simulink model "lookuptable1D"  (Simulink 7.9)
settings: Solver=FixedStepDiscrete  StartTime=0.0  StopTime=10.0  FixedStep=1  RelTol=1e-3
settings Model: Creator=hnine  LastModifiedBy=hnine

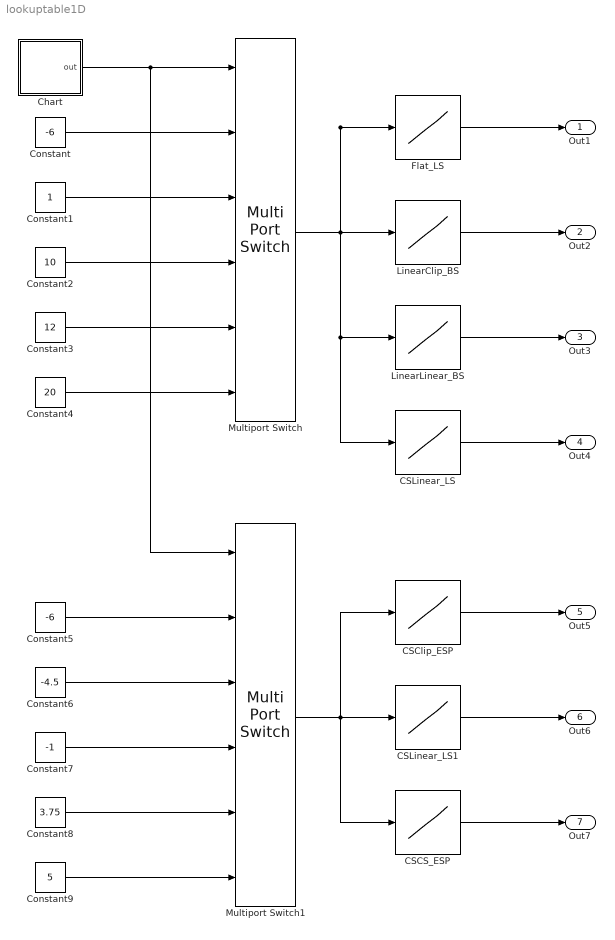
== system lookuptable1D ==
  CSCS_ESP : Lookup_n-D  NumberOfTableDimensions=1  BreakpointsForDimension1=[ -5 -4 -3 -2 -1 0 1 2 3 4 ]  IndexSearchMethod=Evenly spaced points  Table=[ 10 1 9 2 8 3 7 4 6 5 ]  InterpMethod=Cubic spline  ExtrapMethod=Cubic spline  RndMeth=Simplest  InputSameDT=on
  CSClip_ESP : Lookup_n-D  NumberOfTableDimensions=1  BreakpointsForDimension1=[ -5 -4 -3 -2 -1 0 1 2 3 4 ]  IndexSearchMethod=Evenly spaced points  Table=[ 10 1 9 2 8 3 7 4 6 5 ]  InterpMethod=Cubic spline  ExtrapMethod=Clip  RndMeth=Simplest  InputSameDT=on
  CSLinear_LS : Lookup_n-D  NumberOfTableDimensions=1  BreakpointsForDimension1=[ -4 -2 -0.5 .75 3 8 10 11 11.5 15 ]  IndexSearchMethod=Linear search  Table=[ 10 1 9 2 8 3 7 4 6 5 ]  InterpMethod=Cubic spline  RndMeth=Simplest  InputSameDT=on
  CSLinear_LS1 : Lookup_n-D  NumberOfTableDimensions=1  BreakpointsForDimension1=[ -5 -4 -3 -2 -1 0 1 2 3 4 ]  IndexSearchMethod=Linear search  Table=[ 10 1 9 2 8 3 7 4 6 5 ]  InterpMethod=Cubic spline  RndMeth=Simplest  InputSameDT=on
  Chart : Stateflow chart  TreatAsAtomicUnit=on
  Constant : Constant  Value=-6
  Constant1 : Constant
  Constant2 : Constant  Value=10
  Constant3 : Constant  Value=12
  Constant4 : Constant  Value=20
  Constant5 : Constant  Value=-6
  Constant6 : Constant  Value=-4.5
  Constant7 : Constant  Value=-1
  Constant8 : Constant  Value=3.75
  Constant9 : Constant  Value=5
  Flat_LS : Lookup_n-D  NumberOfTableDimensions=1  BreakpointsForDimension1=[ -4 -2 -0.5 .75 3 8 10 11 11.5 15 ]  IndexSearchMethod=Linear search  Table=[ 10 1 9 2 8 3 7 4 6 5 ]  InterpMethod=Flat  RndMeth=Simplest  InputSameDT=on
  LinearClip_BS : Lookup_n-D  NumberOfTableDimensions=1  BreakpointsForDimension1=[ -4 -2 -0.5 .75 3 8 10 11 11.5 15 ]  Table=[ 10 1 9 2 8 3 7 4 6 5 ]  ExtrapMethod=Clip  RndMeth=Simplest  InputSameDT=on
  LinearLinear_BS : Lookup_n-D  NumberOfTableDimensions=1  BreakpointsForDimension1=[ -4 -2 -0.5 .75 3 8 10 11 11.5 15 ]  Table=[ 10 1 9 2 8 3 7 4 6 5 ]  RndMeth=Simplest  InputSameDT=on
  Multiport Switch : MultiPortSwitch  DataPortOrder=Zero-based contiguous  Inputs=5  DiagnosticForDefault=None  zeroidx=on
  Multiport Switch1 : MultiPortSwitch  DataPortOrder=Zero-based contiguous  Inputs=5  DiagnosticForDefault=None  zeroidx=on
  Out1 : Outport
  Out2 : Outport  Port=2
  Out3 : Outport  Port=3
  Out4 : Outport  Port=4
  Out5 : Outport  Port=5
  Out6 : Outport  Port=6
  Out7 : Outport  Port=7
  wires:
  Flat_LS/1 -> Out1/1
  Chart/1(out) -> Multiport Switch/1, Multiport Switch1/1
  Constant/1 -> Multiport Switch/2
  Constant1/1 -> Multiport Switch/3
  Constant2/1 -> Multiport Switch/4
  Constant3/1 -> Multiport Switch/5
  Constant4/1 -> Multiport Switch/6
  LinearClip_BS/1 -> Out2/1
  LinearLinear_BS/1 -> Out3/1
  CSClip_ESP/1 -> Out5/1
  CSLinear_LS/1 -> Out4/1
  CSCS_ESP/1 -> Out7/1
  Multiport Switch/1 -> Flat_LS/1, LinearClip_BS/1, LinearLinear_BS/1, CSLinear_LS/1
  Constant5/1 -> Multiport Switch1/2
  Constant6/1 -> Multiport Switch1/3
  Constant7/1 -> Multiport Switch1/4
  Constant8/1 -> Multiport Switch1/5
  Constant9/1 -> Multiport Switch1/6
  Multiport Switch1/1 -> CSClip_ESP/1, CSCS_ESP/1, CSLinear_LS1/1
  CSLinear_LS1/1 -> Out6/1

== stateflow chart Chart ==
  state count
    en: out = 0;
    du: out = out + 1;
  (default) -> count
  count -> count : [ out >= 4 ]
  data: out output double =0
